simulink model "IP_Core_SS_Switch_and_PWM"  (R2021a)
settings: Solver=VariableStepAuto  StartTime=0.0  StopTime=0.05  RelTol=1e-3
undefined symbols (not defined in the file): f_FPGA_clk, T_FPGA_clk
libraries: hdlsllib x2
(part 1 of 2)
settings Model: Creator=BHK  LastModifiedBy=hoernermi
settings SolverCC: AlgebraicLoopSolver=TrustRegion
settings DataIOCC: ReturnWorkspaceOutputs=off
settings OptimizationCC: BlockReduction=off  ConditionallyExecuteInputs=off  DefaultParameterBehavior=Inlined
settings DebuggingCC: AlgebraicLoopMsg=error  SFMachineParentedDataDiag=warning  ArithmeticOperatorsInVariantConditions=warning
settings HardwareCC: ProdBitPerPointer=32  ProdBitPerSizeT=32  ProdBitPerPtrDiffT=32  ProdLargestAtomicFloat=None  ProdIntDivRoundTo=Undefined  ProdEndianess=Unspecified  ProdWordSize=32  ProdHWDeviceType=ASIC/FPGA->ASIC/FPGA  TargetBitPerPointer=64  TargetBitPerSizeT=64  TargetBitPerPtrDiffT=64  TargetLongLongMode=on  TargetIntDivRoundTo=Zero  TargetEndianess=LittleEndian  TargetWordSize=64  TargetHWDeviceType=Custom Processor->MATLAB Host Computer  ProdEqTarget=off
settings SFSimCC: SimUseLocalCustomCode=off  CustomCodeUndefinedFunction=UseInterfaceOnly
settings RTWCC: RTWUseLocalCustomCode=off

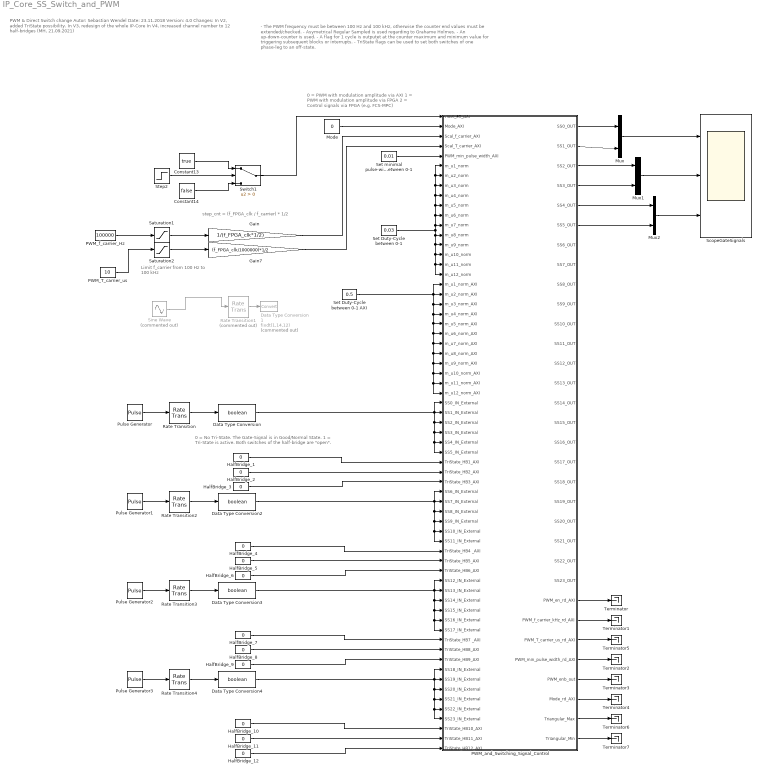
== system IP_Core_SS_Switch_and_PWM ==
  note: 0 = No Tri-State. The Gate-Signal is in Good/Normal State.
      | 1 = Tri-State is active. Both switches of the half-bridge are "open".
  note: PWM & Direct Switch change
      |
      | Autor: Sebastian Wendel
      | Date: 23.11.2018
      | Version: 4.0
      | Changes: In V2, added TriState possibility.
      | In V3, redesign of the whole IP-Core
      | In V4, increased channel number to 12
      | half-bridges (MH, 21.09.2021)
  note: 0 = PWM with modulation amplitude via AXI
      | 1 = PWM with modulation amplitude via FPGA
      | 2 = Control signals via FPGA (e.g. FCS-MPC)
  note: step_cnt = (f_FPGA_clk / f_carrier) * 1/2
  note: Limit f_carrier from
      | 100 Hz to 100 kHz
  note: - The PWM frequency must be between 100 Hz and 100 kHz, otherwise the counter end values must be extended/checked.
      | - Asymetrical Regular Sampled is used regarding to Grahame Holmes.
      | - An up-down-counter is used.
      | - A flag for 1 cycle is outputet at the counter maximum and minimum value for triggering subsequent blocks or interrupts.
      | - TriState flags can be used to set both switches of one phase-leg to an off-state.
  Constant13 : Constant  Value=true  SampleTime=T_FPGA_clk
  Constant14 : Constant  Value=false  SampleTime=T_FPGA_clk
  Data Type Conversion{,2..4} (4 alike) : DataTypeConversion  OutDataTypeStr=boolean
  Data Type Conversion1 : DataTypeConversion  Commented=on  OutDataTypeStr=fixdt(1,14,12)
  Gain : Gain  Gain=1/(f_FPGA_clk*1/2)  OutDataTypeStr=fixdt(0,25,26)
  Gain7 : Gain  Gain=(f_FPGA_clk/1000000)*1/2  OutDataTypeStr=fixdt(0,25,0)
  HalfBridge_{1..12} (12 alike) : Constant  Value=0  OutDataTypeStr=fixdt(0,2,0)  SampleTime=T_FPGA_clk
  Mode : Constant  Value=0  OutDataTypeStr=fixdt(0,2,0)  SampleTime=T_FPGA_clk
  Mux : Mux  Inputs=2
  Mux1 : Mux  Inputs=2
  Mux2 : Mux  Inputs=2
  PWM_T_carrier_us : Constant  Value=10  OutDataTypeStr=uint32  SampleTime=T_FPGA_clk
  PWM_and_Switching_Signal_Control : Subsystem  TreatAsAtomicUnit=on
  PWM_f_carrier_Hz : Constant  Value=100000  OutDataTypeStr=uint32  SampleTime=T_FPGA_clk
  Pulse Generator{,1..3} (4 alike) : DiscretePulseGenerator  PulseType=Time based  Period=0.01  PulseWidth=5
  Rate Transition{,2..4} (4 alike) : RateTransition  OutPortSampleTime=T_FPGA_clk
  Rate Transition1 : RateTransition  Commented=on  OutPortSampleTime=T_FPGA_clk
  Saturation1 : Saturate  UpperLimit=100000  LowerLimit=100
  Saturation2 : Saturate  UpperLimit=10000  LowerLimit=10
  ScopeGateSignals : Scope  NumInputPorts=3
  Set Duty-Cycle between 0-1 : Constant  Value=0.03  OutDataTypeStr=fixdt(1,14,12)  SampleTime=T_FPGA_clk
  Set Duty-Cycle between 0-1 AXI : Constant  Value=0.5  OutDataTypeStr=fixdt(1,14,12)  SampleTime=T_FPGA_clk
  Set minimal pulse-width between 0-1 : Constant  Value=0.01  OutDataTypeStr=fixdt(1,18,16)  SampleTime=T_FPGA_clk
  Sine Wave : Sin  Commented=on  Frequency=500  SampleTime=0
  Step2 : Step  Time=0.002  SampleTime=T_FPGA_clk
  Switch1 : Switch  Criteria=u2 > Threshold
  Terminator{,1..7} (8 alike) : Terminator
  wires:
  Step2/1 -> Switch1/2
  Constant13/1 -> Switch1/1
  Constant14/1 -> Switch1/3
  Switch1/1 -> PWM_and_Switching_Signal_Control/1(PWM_en_AXI)
  Mode/1 -> PWM_and_Switching_Signal_Control/2(Mode_AXI)
  PWM_f_carrier_Hz/1 -> Saturation1/1
  Set minimal pulse-width between 0-1/1 -> PWM_and_Switching_Signal_Control/5(PWM_min_pulse_width_AXI)
  Sine Wave/1 -> Rate Transition1/1
  PWM_and_Switching_Signal_Control/25(PWM_en_rd_AXI) -> Terminator/1
  PWM_and_Switching_Signal_Control/26(PWM_f_carrier_kHz_rd_AXI) -> Terminator1/1
  PWM_and_Switching_Signal_Control/28(PWM_min_pulse_width_rd_AXI) -> Terminator2/1
  PWM_and_Switching_Signal_Control/29(PWM_enb_out) -> Terminator3/1
  PWM_and_Switching_Signal_Control/30(Mode_rd_AXI) -> Terminator4/1
  Set Duty-Cycle between 0-1 AXI/1 -> PWM_and_Switching_Signal_Control/22(m_u5_norm_AXI), PWM_and_Switching_Signal_Control/29(m_u12_norm_AXI), PWM_and_Switching_Signal_Control/28(m_u11_norm_AXI), PWM_and_Switching_Signal_Control/27(m_u10_norm_AXI), PWM_and_Switching_Signal_Control/26(m_u9_norm_AXI), PWM_and_Switching_Signal_Control/25(m_u8_norm_AXI), PWM_and_Switching_Signal_Control/24(m_u7_norm_AXI), PWM_and_Switching_Signal_Control/23(m_u6_norm_AXI), PWM_and_Switching_Signal_Control/21(m_u4_norm_AXI), PWM_and_Switching_Signal_Control/20(m_u3_norm_AXI), PWM_and_Switching_Signal_Control/18(m_u1_norm_AXI), PWM_and_Switching_Signal_Control/19(m_u2_norm_AXI)
  PWM_and_Switching_Signal_Control/1(SS0_OUT) -> Mux/1
  PWM_and_Switching_Signal_Control/2(SS1_OUT) -> Mux/2
  Mux/1 -> ScopeGateSignals/1
  PWM_and_Switching_Signal_Control/3(SS2_OUT) -> Mux1/1
  PWM_and_Switching_Signal_Control/4(SS3_OUT) -> Mux1/2
  PWM_and_Switching_Signal_Control/5(SS4_OUT) -> Mux2/1
  PWM_and_Switching_Signal_Control/6(SS5_OUT) -> Mux2/2
  Mux2/1 -> ScopeGateSignals/3
  Mux1/1 -> ScopeGateSignals/2
  Data Type Conversion/1 -> PWM_and_Switching_Signal_Control/30(SS0_IN_External), PWM_and_Switching_Signal_Control/34(SS4_IN_External), PWM_and_Switching_Signal_Control/35(SS5_IN_External), PWM_and_Switching_Signal_Control/33(SS3_IN_External), PWM_and_Switching_Signal_Control/32(SS2_IN_External), PWM_and_Switching_Signal_Control/31(SS1_IN_External)
  PWM_T_carrier_us/1 -> Saturation2/1
  Rate Transition/1 -> Data Type Conversion/1
  Pulse Generator/1 -> Rate Transition/1
  PWM_and_Switching_Signal_Control/27(PWM_T_carrier_us_rd_AXI) -> Terminator5/1
  PWM_and_Switching_Signal_Control/31(Triangular_Max) -> Terminator6/1
  HalfBridge_3/1 -> PWM_and_Switching_Signal_Control/38(TriState_HB3_AXI)
  HalfBridge_2/1 -> PWM_and_Switching_Signal_Control/37(TriState_HB2_AXI)
  HalfBridge_1/1 -> PWM_and_Switching_Signal_Control/36(TriState_HB1_AXI)
  PWM_and_Switching_Signal_Control/32(Triangular_Min) -> Terminator7/1
  Gain/1 -> PWM_and_Switching_Signal_Control/3(Scal_f_carrier_AXI)
  Gain7/1 -> PWM_and_Switching_Signal_Control/4(Scal_T_carrier_AXI)
  Saturation1/1 -> Gain/1
  Saturation2/1 -> Gain7/1
  Rate Transition1/1 -> Data Type Conversion1/1
  Set Duty-Cycle between 0-1/1 -> PWM_and_Switching_Signal_Control/6(m_u1_norm), PWM_and_Switching_Signal_Control/7(m_u2_norm), PWM_and_Switching_Signal_Control/8(m_u3_norm), PWM_and_Switching_Signal_Control/9(m_u4_norm), PWM_and_Switching_Signal_Control/10(m_u5_norm), PWM_and_Switching_Signal_Control/11(m_u6_norm), PWM_and_Switching_Signal_Control/12(m_u7_norm), PWM_and_Switching_Signal_Control/17(m_u12_norm), PWM_and_Switching_Signal_Control/16(m_u11_norm), PWM_and_Switching_Signal_Control/15(m_u10_norm), PWM_and_Switching_Signal_Control/14(m_u9_norm), PWM_and_Switching_Signal_Control/13(m_u8_norm)
  HalfBridge_5/1 -> PWM_and_Switching_Signal_Control/46(TriState_HB5_AXI)
  HalfBridge_6/1 -> PWM_and_Switching_Signal_Control/47(TriState_HB6_AXI)
  HalfBridge_4/1 -> PWM_and_Switching_Signal_Control/45(TriState_HB4	_AXI)
  HalfBridge_8/1 -> PWM_and_Switching_Signal_Control/55(TriState_HB8_AXI)
  HalfBridge_9/1 -> PWM_and_Switching_Signal_Control/56(TriState_HB9_AXI)
  HalfBridge_7/1 -> PWM_and_Switching_Signal_Control/54(TriState_HB7	_AXI)
  HalfBridge_11/1 -> PWM_and_Switching_Signal_Control/64(TriState_HB11_AXI)
  HalfBridge_12/1 -> PWM_and_Switching_Signal_Control/65(TriState_HB12_AXI)
  HalfBridge_10/1 -> PWM_and_Switching_Signal_Control/63(TriState_HB10_AXI)
  Rate Transition2/1 -> Data Type Conversion2/1
  Pulse Generator1/1 -> Rate Transition2/1
  Data Type Conversion2/1 -> PWM_and_Switching_Signal_Control/40(SS7_IN_External), PWM_and_Switching_Signal_Control/39(SS6_IN_External), PWM_and_Switching_Signal_Control/41(SS8_IN_External), PWM_and_Switching_Signal_Control/42(SS9_IN_External), PWM_and_Switching_Signal_Control/43(SS10_IN_External), PWM_and_Switching_Signal_Control/44(SS11_IN_External)
  Rate Transition3/1 -> Data Type Conversion3/1
  Pulse Generator2/1 -> Rate Transition3/1
  Data Type Conversion3/1 -> PWM_and_Switching_Signal_Control/48(SS12_IN_External), PWM_and_Switching_Signal_Control/49(SS13_IN_External), PWM_and_Switching_Signal_Control/50(SS14_IN_External), PWM_and_Switching_Signal_Control/51(SS15_IN_External), PWM_and_Switching_Signal_Control/53(SS17_IN_External), PWM_and_Switching_Signal_Control/52(SS16_IN_External)
  Rate Transition4/1 -> Data Type Conversion4/1
  Pulse Generator3/1 -> Rate Transition4/1
  Data Type Conversion4/1 -> PWM_and_Switching_Signal_Control/58(SS19_IN_External), PWM_and_Switching_Signal_Control/57(SS18_IN_External), PWM_and_Switching_Signal_Control/59(SS20_IN_External), PWM_and_Switching_Signal_Control/60(SS21_IN_External), PWM_and_Switching_Signal_Control/61(SS22_IN_External), PWM_and_Switching_Signal_Control/62(SS23_IN_External)

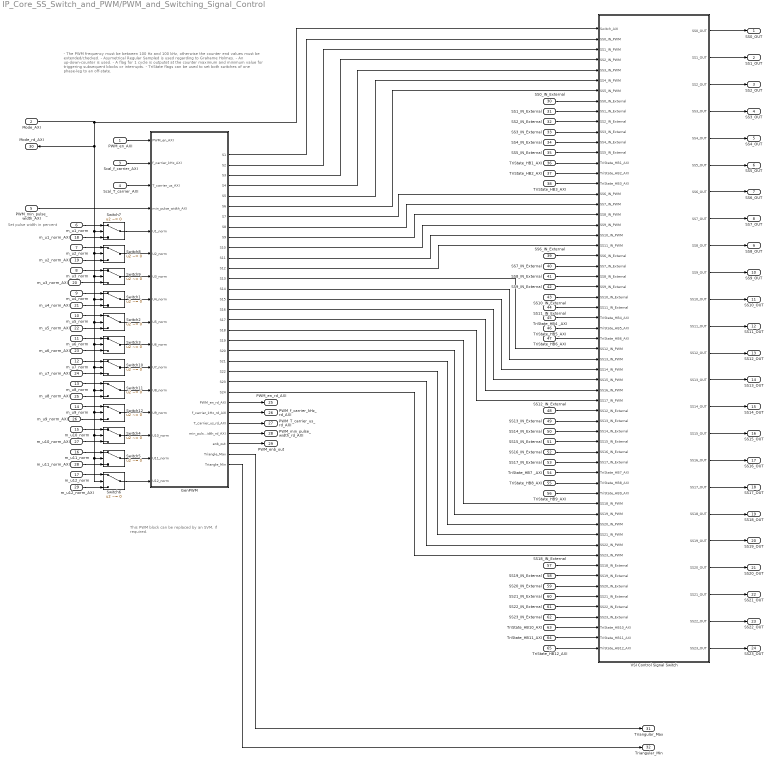
== system IP_Core_SS_Switch_and_PWM/PWM_and_Switching_Signal_Control ==
  note: This PWM block can be replaced by an SVM,
      | if required.
  note: - The PWM frequency must be between 100 Hz and 100 kHz, otherwise the counter end values must be extended/checked.
      | - Asymetrical Regular Sampled is used regarding to Grahame Holmes.
      | - An up-down-counter is used.
      | - A flag for 1 cycle is outputet at the counter maximum and minimum value for triggering subsequent blocks or interrupts.
      | - TriState flags can be used to set both switches of one phase-leg to an off-state.
  note: Set pulse width in percent
  PWM_en_AXI : Inport
  Mode_AXI : Inport  Port=2
  Scal_f_carrier_AXI : Inport  Port=3
  Scal_T_carrier_AXI : Inport  Port=4
  PWM_min_pulse_width_AXI : Inport  Port=5
  m_u1_norm : Inport  Port=6
  m_u2_norm : Inport  Port=7
  m_u3_norm : Inport  Port=8
  m_u4_norm : Inport  Port=9
  m_u5_norm : Inport  Port=10
  m_u6_norm : Inport  Port=11
  m_u7_norm : Inport  Port=12
  m_u8_norm : Inport  Port=13
  m_u9_norm : Inport  Port=14
  m_u10_norm : Inport  Port=15
  m_u11_norm : Inport  Port=16
  m_u12_norm : Inport  Port=17
  m_u1_norm_AXI : Inport  Port=18
  m_u2_norm_AXI : Inport  Port=19
  m_u3_norm_AXI : Inport  Port=20
  m_u4_norm_AXI : Inport  Port=21
  m_u5_norm_AXI : Inport  Port=22
  m_u6_norm_AXI : Inport  Port=23
  m_u7_norm_AXI : Inport  Port=24
  m_u8_norm_AXI : Inport  Port=25
  m_u9_norm_AXI : Inport  Port=26
  m_u10_norm_AXI : Inport  Port=27
  m_u11_norm_AXI : Inport  Port=28
  m_u12_norm_AXI : Inport  Port=29
  SS0_IN_External : Inport  Port=30
  SS1_IN_External : Inport  Port=31
  SS2_IN_External : Inport  Port=32
  SS3_IN_External : Inport  Port=33
  SS4_IN_External : Inport  Port=34
  SS5_IN_External : Inport  Port=35
  TriState_HB1_AXI : Inport  Port=36
  TriState_HB2_AXI : Inport  Port=37
  TriState_HB3_AXI : Inport  Port=38
  SS6_IN_External : Inport  Port=39
  SS7_IN_External : Inport  Port=40
  SS8_IN_External : Inport  Port=41
  SS9_IN_External : Inport  Port=42
  SS10_IN_External : Inport  Port=43
  SS11_IN_External : Inport  Port=44
  TriState_HB4	_AXI : Inport  Port=45
  TriState_HB5_AXI : Inport  Port=46
  TriState_HB6_AXI : Inport  Port=47
  SS12_IN_External : Inport  Port=48
  SS13_IN_External : Inport  Port=49
  SS14_IN_External : Inport  Port=50
  SS15_IN_External : Inport  Port=51
  SS16_IN_External : Inport  Port=52
  SS17_IN_External : Inport  Port=53
  TriState_HB7	_AXI : Inport  Port=54
  TriState_HB8_AXI : Inport  Port=55
  TriState_HB9_AXI : Inport  Port=56
  SS18_IN_External : Inport  Port=57
  SS19_IN_External : Inport  Port=58
  SS20_IN_External : Inport  Port=59
  SS21_IN_External : Inport  Port=60
  SS22_IN_External : Inport  Port=61
  SS23_IN_External : Inport  Port=62
  TriState_HB10_AXI : Inport  Port=63
  TriState_HB11_AXI : Inport  Port=64
  TriState_HB12_AXI : Inport  Port=65
  GenPWM : Subsystem  TreatAsAtomicUnit=on
  Switch{1..12} (12 alike) : Switch  Criteria=u2 ~= 0
  VSI Control Signal Switch : Subsystem
  SS0_OUT : Outport  VectorParamsAs1DForOutWhenUnconnected=off
  SS1_OUT : Outport  Port=2  VectorParamsAs1DForOutWhenUnconnected=off
  SS2_OUT : Outport  Port=3  VectorParamsAs1DForOutWhenUnconnected=off
  SS3_OUT : Outport  Port=4  VectorParamsAs1DForOutWhenUnconnected=off
  SS4_OUT : Outport  Port=5  VectorParamsAs1DForOutWhenUnconnected=off
  SS5_OUT : Outport  Port=6  VectorParamsAs1DForOutWhenUnconnected=off
  SS6_OUT : Outport  Port=7  VectorParamsAs1DForOutWhenUnconnected=off
  SS7_OUT : Outport  Port=8  VectorParamsAs1DForOutWhenUnconnected=off
  SS8_OUT : Outport  Port=9  VectorParamsAs1DForOutWhenUnconnected=off
  SS9_OUT : Outport  Port=10  VectorParamsAs1DForOutWhenUnconnected=off
  SS10_OUT : Outport  Port=11  VectorParamsAs1DForOutWhenUnconnected=off
  SS11_OUT : Outport  Port=12  VectorParamsAs1DForOutWhenUnconnected=off
  SS12_OUT : Outport  Port=13  VectorParamsAs1DForOutWhenUnconnected=off
  SS13_OUT : Outport  Port=14  VectorParamsAs1DForOutWhenUnconnected=off
  SS14_OUT : Outport  Port=15  VectorParamsAs1DForOutWhenUnconnected=off
  SS15_OUT : Outport  Port=16  VectorParamsAs1DForOutWhenUnconnected=off
  SS16_OUT : Outport  Port=17  VectorParamsAs1DForOutWhenUnconnected=off
  SS17_OUT : Outport  Port=18  VectorParamsAs1DForOutWhenUnconnected=off
  SS18_OUT : Outport  Port=19  VectorParamsAs1DForOutWhenUnconnected=off
  SS19_OUT : Outport  Port=20  VectorParamsAs1DForOutWhenUnconnected=off
  SS20_OUT : Outport  Port=21  VectorParamsAs1DForOutWhenUnconnected=off
  SS21_OUT : Outport  Port=22  VectorParamsAs1DForOutWhenUnconnected=off
  SS22_OUT : Outport  Port=23  VectorParamsAs1DForOutWhenUnconnected=off
  SS23_OUT : Outport  Port=24  VectorParamsAs1DForOutWhenUnconnected=off
  PWM_en_rd_AXI : Outport  Port=25  VectorParamsAs1DForOutWhenUnconnected=off
  PWM_f_carrier_kHz_rd_AXI : Outport  Port=26  VectorParamsAs1DForOutWhenUnconnected=off
  PWM_T_carrier_us_rd_AXI : Outport  Port=27  VectorParamsAs1DForOutWhenUnconnected=off
  PWM_min_pulse_width_rd_AXI : Outport  Port=28  VectorParamsAs1DForOutWhenUnconnected=off
  PWM_enb_out : Outport  Port=29  VectorParamsAs1DForOutWhenUnconnected=off
  Mode_rd_AXI : Outport  Port=30  VectorParamsAs1DForOutWhenUnconnected=off
  Triangular_Max : Outport  Port=31  VectorParamsAs1DForOutWhenUnconnected=off
  Triangular_Min : Outport  Port=32  VectorParamsAs1DForOutWhenUnconnected=off
  wires:
  VSI Control Signal Switch/1(SS0_OUT) -> SS0_OUT/1
  GenPWM/4(S4) -> VSI Control Signal Switch/5(SS3_IN_PWM)
  Scal_f_carrier_AXI/1 -> GenPWM/2(f_carrier_kHz_AXI)
  GenPWM/2(S2) -> VSI Control Signal Switch/3(SS1_IN_PWM)
  SS1_IN_External/1 -> VSI Control Signal Switch/9(SS1_IN_External)
  GenPWM/3(S3) -> VSI Control Signal Switch/4(SS2_IN_PWM)
  GenPWM/5(S5) -> VSI Control Signal Switch/6(SS4_IN_PWM)
  GenPWM/6(S6) -> VSI Control Signal Switch/7(SS5_IN_PWM)
  VSI Control Signal Switch/6(SS5_OUT) -> SS5_OUT/1
  GenPWM/1(S1) -> VSI Control Signal Switch/2(SS0_IN_PWM)
  GenPWM/29(enb_out) -> PWM_enb_out/1
  VSI Control Signal Switch/3(SS2_OUT) -> SS2_OUT/1
  SS3_IN_External/1 -> VSI Control Signal Switch/11(SS3_IN_External)
  SS0_IN_External/1 -> VSI Control Signal Switch/8(SS0_IN_External)
  VSI Control Signal Switch/2(SS1_OUT) -> SS1_OUT/1
  SS4_IN_External/1 -> VSI Control Signal Switch/12(SS4_IN_External)
  PWM_en_AXI/1 -> GenPWM/1(PWM_en_AXI)
  SS5_IN_External/1 -> VSI Control Signal Switch/13(SS5_IN_External)
  VSI Control Signal Switch/5(SS4_OUT) -> SS4_OUT/1
  PWM_min_pulse_width_AXI/1 -> GenPWM/4(min_pulse_width_AXI)
  SS2_IN_External/1 -> VSI Control Signal Switch/10(SS2_IN_External)
  VSI Control Signal Switch/4(SS3_OUT) -> SS3_OUT/1
  Switch9/1 -> GenPWM/7(U3_norm)
  m_u1_norm_AXI/1 -> Switch7/3
  m_u1_norm/1 -> Switch7/1
  m_u2_norm/1 -> Switch8/1
  m_u2_norm_AXI/1 -> Switch8/3
  m_u3_norm/1 -> Switch9/1
  m_u3_norm_AXI/1 -> Switch9/3
  GenPWM/25(PWM_en_rd_AXI) -> PWM_en_rd_AXI/1
  GenPWM/26(f_carrier_kHz_rd_AXI) -> PWM_f_carrier_kHz_rd_AXI/1
  GenPWM/28(min_pulse_width_rd_AXI) -> PWM_min_pulse_width_rd_AXI/1
  GenPWM/27(T_carrier_us_rd_AXI) -> PWM_T_carrier_us_rd_AXI/1
  Switch8/1 -> GenPWM/6(U2_norm)
  Switch7/1 -> GenPWM/5(U1_norm)
  Scal_T_carrier_AXI/1 -> GenPWM/3(T_carrier_us_AXI)
  GenPWM/30(Triangle_Max) -> Triangular_Max/1
  TriState_HB1_AXI/1 -> VSI Control Signal Switch/14(TriState_HB1_AXI)
  TriState_HB2_AXI/1 -> VSI Control Signal Switch/15(TriState_HB2_AXI)
  TriState_HB3_AXI/1 -> VSI Control Signal Switch/16(TriState_HB3_AXI)
  GenPWM/31(Triangle_Min) -> Triangular_Min/1
  GenPWM/7(S7) -> VSI Control Signal Switch/17(SS6_IN_PWM)
  GenPWM/8(S8) -> VSI Control Signal Switch/18(SS7_IN_PWM)
  GenPWM/9(S9) -> VSI Control Signal Switch/19(SS8_IN_PWM)
  GenPWM/10(S10) -> VSI Control Signal Switch/20(SS9_IN_PWM)
  GenPWM/11(S11) -> VSI Control Signal Switch/21(SS10_IN_PWM)
  GenPWM/12(S12) -> VSI Control Signal Switch/22(SS11_IN_PWM)
  SS6_IN_External/1 -> VSI Control Signal Switch/23(SS6_IN_External)
  TriState_HB6_AXI/1 -> VSI Control Signal Switch/31(TriState_HB6_AXI)
  SS10_IN_External/1 -> VSI Control Signal Switch/27(SS10_IN_External)
  TriState_HB5_AXI/1 -> VSI Control Signal Switch/30(TriState_HB5_AXI)
  SS11_IN_External/1 -> VSI Control Signal Switch/28(SS11_IN_External)
  SS8_IN_External/1 -> VSI Control Signal Switch/25(SS8_IN_External)
  SS9_IN_External/1 -> VSI Control Signal Switch/26(SS9_IN_External)
  SS7_IN_External/1 -> VSI Control Signal Switch/24(SS7_IN_External)
  TriState_HB4	_AXI/1 -> VSI Control Signal Switch/29(TriState_HB4_AXI)
  GenPWM/13(S13) -> VSI Control Signal Switch/32(SS12_IN_PWM)
  GenPWM/14(S14) -> VSI Control Signal Switch/33(SS13_IN_PWM)
  GenPWM/15(S15) -> VSI Control Signal Switch/34(SS14_IN_PWM)
  GenPWM/16(S16) -> VSI Control Signal Switch/35(SS15_IN_PWM)
  GenPWM/17(S17) -> VSI Control Signal Switch/36(SS16_IN_PWM)
  GenPWM/18(S18) -> VSI Control Signal Switch/37(SS17_IN_PWM)
  SS16_IN_External/1 -> VSI Control Signal Switch/42(SS16_IN_External)
  SS14_IN_External/1 -> VSI Control Signal Switch/40(SS14_IN_External)
  SS13_IN_External/1 -> VSI Control Signal Switch/39(SS13_IN_External)
  TriState_HB9_AXI/1 -> VSI Control Signal Switch/46(TriState_HB9_AXI)
  SS15_IN_External/1 -> VSI Control Signal Switch/41(SS15_IN_External)
  TriState_HB8_AXI/1 -> VSI Control Signal Switch/45(TriState_HB8_AXI)
  SS12_IN_External/1 -> VSI Control Signal Switch/38(SS12_IN_External)
  SS17_IN_External/1 -> VSI Control Signal Switch/43(SS17_IN_External)
  TriState_HB7	_AXI/1 -> VSI Control Signal Switch/44(TriState_HB7_AXI)
  GenPWM/19(S19) -> VSI Control Signal Switch/47(SS18_IN_PWM)
  GenPWM/20(S20) -> VSI Control Signal Switch/48(SS19_IN_PWM)
  GenPWM/21(S21) -> VSI Control Signal Switch/49(SS20_IN_PWM)
  GenPWM/22(S22) -> VSI Control Signal Switch/50(SS21_IN_PWM)
  GenPWM/23(S23) -> VSI Control Signal Switch/51(SS22_IN_PWM)
  GenPWM/24(S24) -> VSI Control Signal Switch/52(SS23_IN_PWM)
  TriState_HB10_AXI/1 -> VSI Control Signal Switch/59(TriState_HB10_AXI)
  TriState_HB12_AXI/1 -> VSI Control Signal Switch/61(TriState_HB12_AXI)
  SS21_IN_External/1 -> VSI Control Signal Switch/56(SS21_IN_External)
  SS22_IN_External/1 -> VSI Control Signal Switch/57(SS22_IN_External)
  SS23_IN_External/1 -> VSI Control Signal Switch/58(SS23_IN_External)
  SS18_IN_External/1 -> VSI Control Signal Switch/53(SS18_IN_External)
  TriState_HB11_AXI/1 -> VSI Control Signal Switch/60(TriState_HB11_AXI)
  SS20_IN_External/1 -> VSI Control Signal Switch/55(SS20_IN_External)
  SS19_IN_External/1 -> VSI Control Signal Switch/54(SS19_IN_External)
  VSI Control Signal Switch/11(SS10_OUT) -> SS10_OUT/1
  VSI Control Signal Switch/8(SS7_OUT) -> SS7_OUT/1
  VSI Control Signal Switch/7(SS6_OUT) -> SS6_OUT/1
  VSI Control Signal Switch/10(SS9_OUT) -> SS9_OUT/1
  VSI Control Signal Switch/12(SS11_OUT) -> SS11_OUT/1
  VSI Control Signal Switch/9(SS8_OUT) -> SS8_OUT/1
  VSI Control Signal Switch/21(SS20_OUT) -> SS20_OUT/1
  VSI Control Signal Switch/19(SS18_OUT) -> SS18_OUT/1
  VSI Control Signal Switch/22(SS21_OUT) -> SS21_OUT/1
  VSI Control Signal Switch/20(SS19_OUT) -> SS19_OUT/1
  VSI Control Signal Switch/17(SS16_OUT) -> SS16_OUT/1
  VSI Control Signal Switch/14(SS13_OUT) -> SS13_OUT/1
  VSI Control Signal Switch/16(SS15_OUT) -> SS15_OUT/1
  VSI Control Signal Switch/13(SS12_OUT) -> SS12_OUT/1
  VSI Control Signal Switch/23(SS22_OUT) -> SS22_OUT/1
  VSI Control Signal Switch/18(SS17_OUT) -> SS17_OUT/1
  VSI Control Signal Switch/24(SS23_OUT) -> SS23_OUT/1
  VSI Control Signal Switch/15(SS14_OUT) -> SS14_OUT/1
  Switch2/1 -> GenPWM/9(U5_norm)
  m_u5_norm_AXI/1 -> Switch2/3
  Switch3/1 -> GenPWM/10(U6_norm)
  m_u4_norm_AXI/1 -> Switch1/3
  m_u4_norm/1 -> Switch1/1
  m_u6_norm/1 -> Switch3/1
  m_u6_norm_AXI/1 -> Switch3/3
  m_u5_norm/1 -> Switch2/1
  Switch1/1 -> GenPWM/8(U4_norm)
  m_u11_norm/1 -> Switch5/1
  m_u12_norm_AXI/1 -> Switch6/3
  m_u12_norm/1 -> Switch6/1
  m_u10_norm/1 -> Switch4/1
  m_u11_norm_AXI/1 -> Switch5/3
  m_u10_norm_AXI/1 -> Switch4/3
  Switch6/1 -> GenPWM/16(U12_norm)
  Switch5/1 -> GenPWM/15(U11_norm)
  Switch4/1 -> GenPWM/14(U10_norm)
  Switch11/1 -> GenPWM/12(U8_norm)
  m_u8_norm_AXI/1 -> Switch11/3
  Switch12/1 -> GenPWM/13(U9_norm)
  m_u7_norm_AXI/1 -> Switch10/3
  m_u7_norm/1 -> Switch10/1
  m_u9_norm/1 -> Switch12/1
  Mode_AXI/1 -> Mode_rd_AXI/1, Switch1/2, Switch4/2, Switch6/2, Switch5/2, Switch12/2, Switch11/2, Switch10/2, Switch3/2, Switch2/2, Switch9/2, Switch8/2, Switch7/2, VSI Control Signal Switch/1(Switch_AXI)
  m_u9_norm_AXI/1 -> Switch12/3
  m_u8_norm/1 -> Switch11/1
  Switch10/1 -> GenPWM/11(U7_norm)

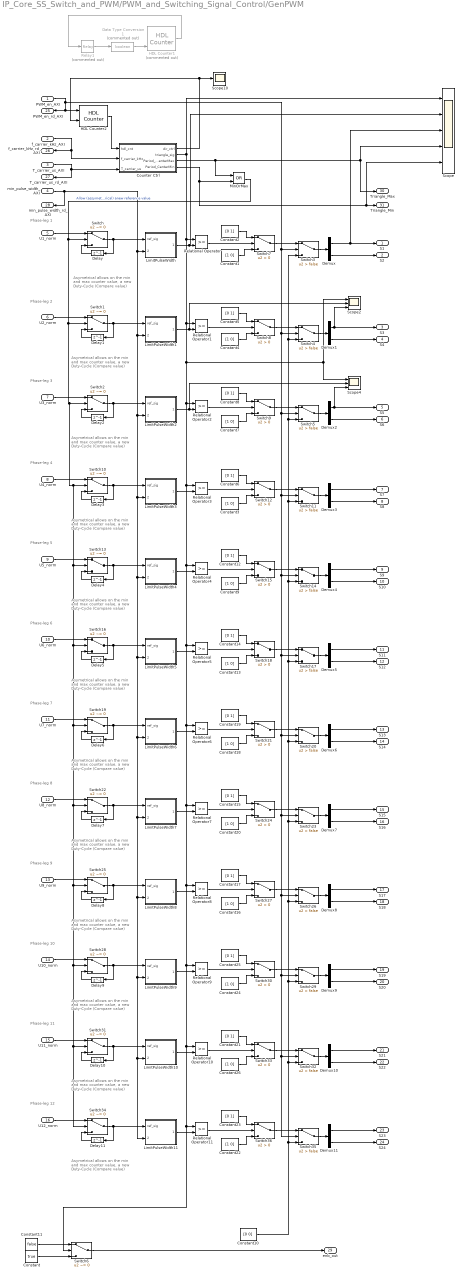
== system IP_Core_SS_Switch_and_PWM/PWM_and_Switching_Signal_Control/GenPWM ==
  note: Asymetrical allows on the min
      |  and max counter value, a new
      |  Duty-Cycle (Compare value)
  note: Phase-leg 1
  note: Phase-leg 2
  note: Phase-leg 3
  note: Asymetrical allows on the min
      |  and max counter value, a new
      |  Duty-Cycle (Compare value)
  note: Asymetrical allows on the min
      |  and max counter value, a new
      |  Duty-Cycle (Compare value)
  note: Phase-leg 4
  note: Asymetrical allows on the min
      |  and max counter value, a new
      |  Duty-Cycle (Compare value)
  note: Phase-leg 5
  note: Asymetrical allows on the min
      |  and max counter value, a new
      |  Duty-Cycle (Compare value)
  note: Phase-leg 6
  note: Asymetrical allows on the min
      |  and max counter value, a new
      |  Duty-Cycle (Compare value)
  note: Asymetrical allows on the min
      |  and max counter value, a new
      |  Duty-Cycle (Compare value)
  note: Phase-leg 9
  note: Asymetrical allows on the min
      |  and max counter value, a new
      |  Duty-Cycle (Compare value)
  note: Phase-leg 8
  note: Asymetrical allows on the min
      |  and max counter value, a new
      |  Duty-Cycle (Compare value)
  note: Phase-leg 7
  note: Asymetrical allows on the min
      |  and max counter value, a new
      |  Duty-Cycle (Compare value)
  note: Phase-leg 12
  note: Asymetrical allows on the min
      |  and max counter value, a new
      |  Duty-Cycle (Compare value)
  note: Phase-leg 11
  note: Asymetrical allows on the min
      |  and max counter value, a new
      |  Duty-Cycle (Compare value)
  note: Phase-leg 10
  PWM_en_AXI : Inport
  f_carrier_kHz_AXI : Inport  Port=2
  T_carrier_us_AXI : Inport  Port=3
  min_pulse_width_AXI : Inport  Port=4
  U1_norm : Inport  Port=5
  U2_norm : Inport  Port=6
  U3_norm : Inport  Port=7
  U4_norm : Inport  Port=8
  U5_norm : Inport  Port=9
  U6_norm : Inport  Port=10
  U7_norm : Inport  Port=11
  U8_norm : Inport  Port=12
  U9_norm : Inport  Port=13
  U10_norm : Inport  Port=14
  U11_norm : Inport  Port=15
  U12_norm : Inport  Port=16
  Constant : Constant  Value=true  SampleTime=T_FPGA_clk
  Constant{1,3..4,7,9,13,16,18,20,22,24,26} (12 alike) : Constant  Value=[1 0]  OutDataTypeStr=fixdt(0,1,0)  SampleTime=T_FPGA_clk
  Constant10 : Constant  Value=[0 0]  OutDataTypeStr=fixdt(0,1,0)  SampleTime=T_FPGA_clk
  Constant11 : Constant  Value=false  SampleTime=T_FPGA_clk
  Constant{2,5..6,8,12,14..15,17,19,21,23,25} (12 alike) : Constant  Value=[0 1]  OutDataTypeStr=fixdt(0,1,0)  SampleTime=T_FPGA_clk
  Counter Ctrl : Subsystem
  Data Type Conversion1 : DataTypeConversion  Commented=on  OutDataTypeStr=boolean
  Delay{,1..11} (12 alike) : Delay  DelayLength=1
  Demux{,1..11} (12 alike) : Demux  Outputs=2
  HDL Counter1 : hdlsllib/Sources/HDL Counter  Commented=on  CountType=Free running  CountInit=0  CountStep=1  CountMax=100  CountFromType=Initial value  CountFrom=0  CountResetPort=on  CountLoadPort=off  CountEnbPort=on  CountDirPort=on  CountHitOutputPort=off  CountDataType=Signed  CountWordLen=8  CountFracLen=0  CountSampTime=Ts
  HDL Counter2 : hdlsllib/Sources/HDL Counter  CountType=Free running  CountInit=0  CountStep=1  CountMax=100  CountFromType=Initial value  CountFrom=0  CountResetPort=off  CountLoadPort=off  CountEnbPort=on  CountDirPort=on  CountHitOutputPort=off  CountDataType=Unsigned  CountWordLen=20  CountFracLen=0  CountSampTime=1
  LimitPulseWidth : Subsystem
  LimitPulseWidth1 : Subsystem
  LimitPulseWidth10 : Subsystem
  LimitPulseWidth11 : Subsystem
  LimitPulseWidth2 : Subsystem
  LimitPulseWidth3 : Subsystem
  LimitPulseWidth4 : Subsystem
  LimitPulseWidth5 : Subsystem
  LimitPulseWidth6 : Subsystem
  LimitPulseWidth7 : Subsystem
  LimitPulseWidth8 : Subsystem
  LimitPulseWidth9 : Subsystem
  MinOrMax : Logic  Operator=OR  AllPortsSameDT=off  OutDataTypeStr=boolean
  Relational Operator{,1..11} (12 alike) : RelationalOperator  OutDataTypeStr=boolean  RndMeth=Nearest
  Relay1 : Relay  Commented=on  OnSwitchValue=100  OffSwitchValue=0  OnOutputValue=0  OffOutputValue=1
  Scope : Scope  NumInputPorts=5
  Scope10 : Scope
  Scope2 : Scope  NumInputPorts=3
  Scope4 : Scope  NumInputPorts=3
  Switch : Switch  Criteria=u2 ~= 0  Threshold=1
  Switch{1..2,6,10,13,16,19,22,25,28,31,34} (12 alike) : Switch  Criteria=u2 ~= 0
  Switch{3..5,11,14,17,20,23,26,29,32,35} (12 alike) : Switch  Criteria=u2 > Threshold  Threshold=false
  Switch{7..9,12,15,18,21,24,27,30,33,36} (12 alike) : Switch  Criteria=u2 > Threshold
  S1 : Outport  VectorParamsAs1DForOutWhenUnconnected=off
  S2 : Outport  Port=2  VectorParamsAs1DForOutWhenUnconnected=off
  S3 : Outport  Port=3  VectorParamsAs1DForOutWhenUnconnected=off
  S4 : Outport  Port=4  VectorParamsAs1DForOutWhenUnconnected=off
  S5 : Outport  Port=5  VectorParamsAs1DForOutWhenUnconnected=off
  S6 : Outport  Port=6  VectorParamsAs1DForOutWhenUnconnected=off
  S7 : Outport  Port=7  VectorParamsAs1DForOutWhenUnconnected=off
  S8 : Outport  Port=8  VectorParamsAs1DForOutWhenUnconnected=off
  S9 : Outport  Port=9  VectorParamsAs1DForOutWhenUnconnected=off
  S10 : Outport  Port=10  VectorParamsAs1DForOutWhenUnconnected=off
  S11 : Outport  Port=11  VectorParamsAs1DForOutWhenUnconnected=off
  S12 : Outport  Port=12  VectorParamsAs1DForOutWhenUnconnected=off
  S13 : Outport  Port=13  VectorParamsAs1DForOutWhenUnconnected=off
  S14 : Outport  Port=14  VectorParamsAs1DForOutWhenUnconnected=off
  S15 : Outport  Port=15  VectorParamsAs1DForOutWhenUnconnected=off
  S16 : Outport  Port=16  VectorParamsAs1DForOutWhenUnconnected=off
  S17 : Outport  Port=17  VectorParamsAs1DForOutWhenUnconnected=off
  S18 : Outport  Port=18  VectorParamsAs1DForOutWhenUnconnected=off
  S19 : Outport  Port=19  VectorParamsAs1DForOutWhenUnconnected=off
  S20 : Outport  Port=20  VectorParamsAs1DForOutWhenUnconnected=off
  S21 : Outport  Port=21  VectorParamsAs1DForOutWhenUnconnected=off
  S22 : Outport  Port=22  VectorParamsAs1DForOutWhenUnconnected=off
  S23 : Outport  Port=23  VectorParamsAs1DForOutWhenUnconnected=off
  S24 : Outport  Port=24  VectorParamsAs1DForOutWhenUnconnected=off
  PWM_en_rd_AXI : Outport  Port=25  VectorParamsAs1DForOutWhenUnconnected=off
  f_carrier_kHz_rd_AXI : Outport  Port=26  VectorParamsAs1DForOutWhenUnconnected=off
  T_carrier_us_rd_AXI : Outport  Port=27  VectorParamsAs1DForOutWhenUnconnected=off
  min_pulse_width_rd_AXI : Outport  Port=28  VectorParamsAs1DForOutWhenUnconnected=off
  enb_out : Outport  Port=29  VectorParamsAs1DForOutWhenUnconnected=off
  Triangle_Max : Outport  Port=30  VectorParamsAs1DForOutWhenUnconnected=off
  Triangle_Min : Outport  Port=31  VectorParamsAs1DForOutWhenUnconnected=off
  wires:
  Constant7/1 -> Switch9/3
  Demux2/2 -> S6/1
  Constant8/1 -> Switch9/1
  Relational Operator2/1 -> Switch9/2
  Switch9/1 -> Switch5/1
  Demux/2 -> S2/1
  Relational Operator/1 -> Switch7/2
  Demux1/2 -> S4/1
  Constant5/1 -> Switch8/1
  Relational Operator1/1 -> Switch8/2
  Constant4/1 -> Switch8/3
  Constant1/1 -> Switch7/3
  Constant2/1 -> Switch7/1
  LimitPulseWidth/1(ref_sig_limit) -> Scope/2, Relational Operator/2
  LimitPulseWidth1/1(ref_sig_limit) -> Scope2/2, Relational Operator1/2
  LimitPulseWidth2/1(ref_sig_limit) -> Scope4/2, Relational Operator2/2
  Delay/1 -> Switch/3
  Delay1/1 -> Switch1/3
  Delay2/1 -> Switch2/3
  Switch5/1 -> Demux2/1
  Switch8/1 -> Switch4/1
  Switch4/1 -> Demux1/1
  Switch3/1 -> Demux/1
  U1_norm/1 -> Switch/1
  U3_norm/1 -> Switch2/1
  U2_norm/1 -> Switch1/1
  Counter Ctrl/1(dir_ctrl) -> HDL Counter2/2, Scope10/1
  HDL Counter2/1 -> Counter Ctrl/1(hdl_cnt)
  f_carrier_kHz_AXI/1 -> f_carrier_kHz_rd_AXI/1, Counter Ctrl/2(f_carrier_kHz)
  Relay1/1 -> Data Type Conversion1/1
  Data Type Conversion1/1 -> HDL Counter1/3
  HDL Counter1/1 -> Relay1/1
  Switch/1 -> Delay/1, LimitPulseWidth/1(ref_sig)
  Switch1/1 -> LimitPulseWidth1/1(ref_sig), Delay1/1
  Switch2/1 -> LimitPulseWidth2/1(ref_sig), Delay2/1
  Demux/1 -> Scope/3, S1/1
  Switch6/1 -> enb_out/1
  Constant11/1 -> Switch6/1
  Constant/1 -> Switch6/3
  Demux1/1 -> Scope2/3, S3/1
  Demux2/1 -> Scope4/3, S5/1
  T_carrier_us_AXI/1 -> T_carrier_us_rd_AXI/1, Counter Ctrl/3(T_carrier_us)
  Switch7/1 -> Switch3/1
  Counter Ctrl/3(Period_CenterMax) -> MinOrMax/1, Triangle_Max/1, Scope/4
  Counter Ctrl/4(Period_CenterMin) -> MinOrMax/2, Scope/5, Triangle_Min/1
  Demux3/1 -> S7/1
  Relational Operator3/1 -> Switch12/2
  Switch10/1 -> LimitPulseWidth3/1(ref_sig), Delay3/1
  Switch11/1 -> Demux3/1
  Delay3/1 -> Switch10/3
  U4_norm/1 -> Switch10/1
  Constant10/1 -> Switch3/3, Switch4/3, Switch5/3, Switch11/3, Switch14/3, Switch17/3, Switch20/3, Switch23/3, Switch26/3, Switch29/3, Switch32/3, Switch35/3
  Constant6/1 -> Switch12/1
  Constant3/1 -> Switch12/3
  Switch12/1 -> Switch11/1
  Demux3/2 -> S8/1
  LimitPulseWidth3/1(ref_sig_limit) -> Relational Operator3/2
  U5_norm/1 -> Switch13/1
  Delay4/1 -> Switch13/3
  LimitPulseWidth4/1(ref_sig_limit) -> Relational Operator4/2
  Switch15/1 -> Switch14/1
  Constant9/1 -> Switch15/3
  Constant12/1 -> Switch15/1
  Counter Ctrl/2(triangle_sig) -> Switch6/2, Relational Operator11/1, Relational Operator10/1, Relational Operator9/1, Relational Operator8/1, Relational Operator7/1, Relational Operator6/1, Relational Operator5/1, Relational Operator4/1, Relational Operator3/1, Relational Operator2/1, Scope2/1, Scope4/1, Relational Operator1/1, Relational Operator/1, Scope/1
  Switch14/1 -> Demux4/1
  Demux4/1 -> S9/1
  Relational Operator4/1 -> Switch15/2
  Switch13/1 -> LimitPulseWidth4/1(ref_sig), Delay4/1
  Demux4/2 -> S10/1
  U6_norm/1 -> Switch16/1
  Delay5/1 -> Switch16/3
  LimitPulseWidth5/1(ref_sig_limit) -> Relational Operator5/2
  Switch18/1 -> Switch17/1
  Constant13/1 -> Switch18/3
  Constant14/1 -> Switch18/1
  Switch17/1 -> Demux5/1
  Demux5/1 -> S11/1
  Relational Operator5/1 -> Switch18/2
  Switch16/1 -> LimitPulseWidth5/1(ref_sig), Delay5/1
  Demux5/2 -> S12/1
  Demux8/2 -> S18/1
  Switch25/1 -> LimitPulseWidth8/1(ref_sig), Delay8/1
  Relational Operator8/1 -> Switch27/2
  Switch26/1 -> Demux8/1
  Demux8/1 -> S17/1
  U7_norm/1 -> Switch19/1
  Constant15/1 -> Switch24/1
  Constant18/1 -> Switch21/3
  Constant19/1 -> Switch21/1
  Switch22/1 -> LimitPulseWidth7/1(ref_sig), Delay7/1
  LimitPulseWidth8/1(ref_sig_limit) -> Relational Operator8/2
  Delay6/1 -> Switch19/3
  Delay7/1 -> Switch22/3
  U8_norm/1 -> Switch22/1
  Constant20/1 -> Switch24/3
  Switch21/1 -> Switch20/1
  LimitPulseWidth7/1(ref_sig_limit) -> Relational Operator7/2
  Switch24/1 -> Switch23/1
  Switch19/1 -> LimitPulseWidth6/1(ref_sig), Delay6/1
  Relational Operator7/1 -> Switch24/2
  Demux6/1 -> S13/1
  Relational Operator6/1 -> Switch21/2
  U9_norm/1 -> Switch25/1
  Delay8/1 -> Switch25/3
  Demux7/2 -> S16/1
  Constant17/1 -> Switch27/1
  Switch20/1 -> Demux6/1
  LimitPulseWidth6/1(ref_sig_limit) -> Relational Operator6/2
  Switch23/1 -> Demux7/1
  Constant16/1 -> Switch27/3
  Switch27/1 -> Switch26/1
  Demux6/2 -> S14/1
  Demux7/1 -> S15/1
  Demux11/2 -> S24/1
  MinOrMax/1 -> Switch1/2, Switch34/2, Switch31/2, Switch28/2, Switch25/2, Switch22/2, Switch19/2, Switch16/2, Switch13/2, Switch10/2, Switch2/2, Switch/2  "Allow (assymetrical) anew reference value"
  min_pulse_width_AXI/1 -> LimitPulseWidth/2(min_pulse_width), LimitPulseWidth4/2(min_pulse_width), LimitPulseWidth11/2(min_pulse_width), LimitPulseWidth10/2(min_pulse_width), LimitPulseWidth9/2(min_pulse_width), LimitPulseWidth8/2(min_pulse_width), LimitPulseWidth7/2(min_pulse_width), LimitPulseWidth6/2(min_pulse_width), LimitPulseWidth5/2(min_pulse_width), LimitPulseWidth3/2(min_pulse_width), LimitPulseWidth2/2(min_pulse_width), LimitPulseWidth1/2(min_pulse_width), min_pulse_width_rd_AXI/1
  Switch34/1 -> LimitPulseWidth11/1(ref_sig), Delay11/1
  Relational Operator11/1 -> Switch36/2
  Switch35/1 -> Demux11/1
  Demux11/1 -> S23/1
  U10_norm/1 -> Switch28/1
  Constant21/1 -> Switch33/1
  Constant24/1 -> Switch30/3
  Constant25/1 -> Switch30/1
  Switch31/1 -> LimitPulseWidth10/1(ref_sig), Delay10/1
  LimitPulseWidth11/1(ref_sig_limit) -> Relational Operator11/2
  Delay9/1 -> Switch28/3
  Delay10/1 -> Switch31/3
  U11_norm/1 -> Switch31/1
  Constant26/1 -> Switch33/3
  Switch30/1 -> Switch29/1
  LimitPulseWidth10/1(ref_sig_limit) -> Relational Operator10/2
  Switch33/1 -> Switch32/1
  Switch28/1 -> LimitPulseWidth9/1(ref_sig), Delay9/1
  Relational Operator10/1 -> Switch33/2
  Demux9/1 -> S19/1
  Relational Operator9/1 -> Switch30/2
  U12_norm/1 -> Switch34/1
  Delay11/1 -> Switch34/3
  PWM_en_AXI/1 -> PWM_en_rd_AXI/1, HDL Counter2/1, Switch35/2, Switch32/2, Switch29/2, Switch26/2, Switch23/2, Switch20/2, Switch17/2, Switch14/2, Switch11/2, Switch5/2, Switch4/2, Switch3/2
  Demux10/2 -> S22/1
  Constant23/1 -> Switch36/1
  Switch29/1 -> Demux9/1
  LimitPulseWidth9/1(ref_sig_limit) -> Relational Operator9/2
  Switch32/1 -> Demux10/1
  Constant22/1 -> Switch36/3
  Switch36/1 -> Switch35/1
  Demux9/2 -> S20/1
  Demux10/1 -> S21/1

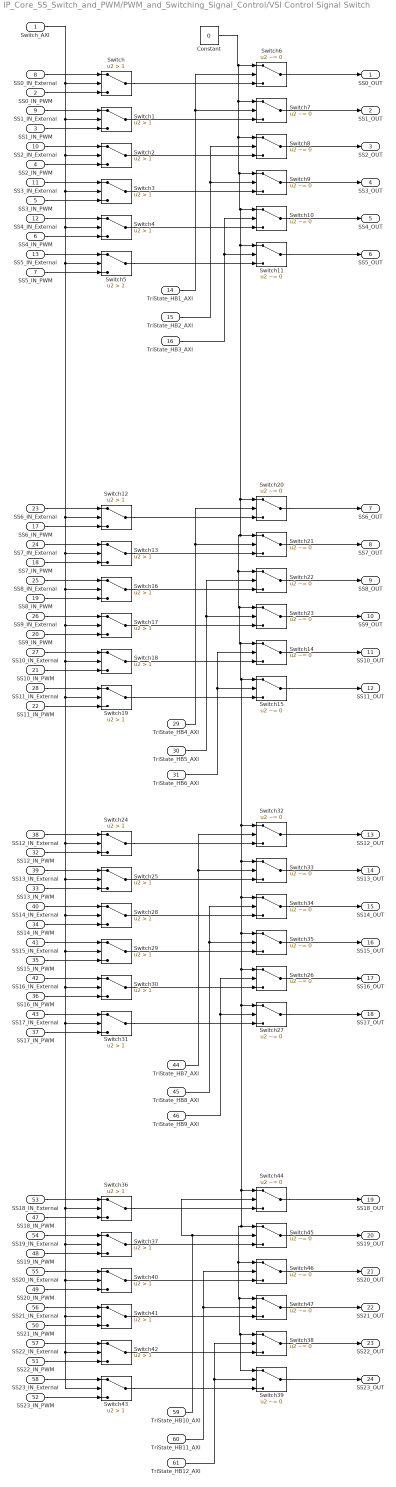
== system IP_Core_SS_Switch_and_PWM/PWM_and_Switching_Signal_Control/VSI Control Signal Switch ==
  Switch_AXI : Inport
  SS0_IN_PWM : Inport  Port=2
  SS1_IN_PWM : Inport  Port=3
  SS2_IN_PWM : Inport  Port=4
  SS3_IN_PWM : Inport  Port=5
  SS4_IN_PWM : Inport  Port=6
  SS5_IN_PWM : Inport  Port=7
  SS0_IN_External : Inport  Port=8
  SS1_IN_External : Inport  Port=9
  SS2_IN_External : Inport  Port=10
  SS3_IN_External : Inport  Port=11
  SS4_IN_External : Inport  Port=12
  SS5_IN_External : Inport  Port=13
  TriState_HB1_AXI : Inport  Port=14
  TriState_HB2_AXI : Inport  Port=15
  TriState_HB3_AXI : Inport  Port=16
  SS6_IN_PWM : Inport  Port=17
  SS7_IN_PWM : Inport  Port=18
  SS8_IN_PWM : Inport  Port=19
  SS9_IN_PWM : Inport  Port=20
  SS10_IN_PWM : Inport  Port=21
  SS11_IN_PWM : Inport  Port=22
  SS6_IN_External : Inport  Port=23
  SS7_IN_External : Inport  Port=24
  SS8_IN_External : Inport  Port=25
  SS9_IN_External : Inport  Port=26
  SS10_IN_External : Inport  Port=27
  SS11_IN_External : Inport  Port=28
  TriState_HB4_AXI : Inport  Port=29
  TriState_HB5_AXI : Inport  Port=30
  TriState_HB6_AXI : Inport  Port=31
  SS12_IN_PWM : Inport  Port=32
  SS13_IN_PWM : Inport  Port=33
  SS14_IN_PWM : Inport  Port=34
  SS15_IN_PWM : Inport  Port=35
  SS16_IN_PWM : Inport  Port=36
  SS17_IN_PWM : Inport  Port=37
  SS12_IN_External : Inport  Port=38
  SS13_IN_External : Inport  Port=39
  SS14_IN_External : Inport  Port=40
  SS15_IN_External : Inport  Port=41
  SS16_IN_External : Inport  Port=42
  SS17_IN_External : Inport  Port=43
  TriState_HB7_AXI : Inport  Port=44
  TriState_HB8_AXI : Inport  Port=45
  TriState_HB9_AXI : Inport  Port=46
  SS18_IN_PWM : Inport  Port=47
  SS19_IN_PWM : Inport  Port=48
  SS20_IN_PWM : Inport  Port=49
  SS21_IN_PWM : Inport  Port=50
  SS22_IN_PWM : Inport  Port=51
  SS23_IN_PWM : Inport  Port=52
  SS18_IN_External : Inport  Port=53
  SS19_IN_External : Inport  Port=54
  SS20_IN_External : Inport  Port=55
  SS21_IN_External : Inport  Port=56
  SS22_IN_External : Inport  Port=57
  SS23_IN_External : Inport  Port=58
  TriState_HB10_AXI : Inport  Port=59
  TriState_HB11_AXI : Inport  Port=60
  TriState_HB12_AXI : Inport  Port=61
  Constant : Constant  Value=0  OutDataTypeStr=boolean  SampleTime=T_FPGA_clk
  Switch{,1..5,12..13,16..19,24..25,28..31,36..37,40..43} (24 alike) : Switch  Criteria=u2 > Threshold  Threshold=1
  Switch{6..11,14..15,20..23,26..27,32..35,38..39,44..47} (24 alike) : Switch  Criteria=u2 ~= 0  Threshold=1
  SS0_OUT : Outport  VectorParamsAs1DForOutWhenUnconnected=off
  SS1_OUT : Outport  Port=2  VectorParamsAs1DForOutWhenUnconnected=off
  SS2_OUT : Outport  Port=3  VectorParamsAs1DForOutWhenUnconnected=off
  SS3_OUT : Outport  Port=4  VectorParamsAs1DForOutWhenUnconnected=off
  SS4_OUT : Outport  Port=5  VectorParamsAs1DForOutWhenUnconnected=off
  SS5_OUT : Outport  Port=6  VectorParamsAs1DForOutWhenUnconnected=off
  SS6_OUT : Outport  Port=7  VectorParamsAs1DForOutWhenUnconnected=off
  SS7_OUT : Outport  Port=8  VectorParamsAs1DForOutWhenUnconnected=off
  SS8_OUT : Outport  Port=9  VectorParamsAs1DForOutWhenUnconnected=off
  SS9_OUT : Outport  Port=10  VectorParamsAs1DForOutWhenUnconnected=off
  SS10_OUT : Outport  Port=11  VectorParamsAs1DForOutWhenUnconnected=off
  SS11_OUT : Outport  Port=12  VectorParamsAs1DForOutWhenUnconnected=off
  SS12_OUT : Outport  Port=13  VectorParamsAs1DForOutWhenUnconnected=off
  SS13_OUT : Outport  Port=14  VectorParamsAs1DForOutWhenUnconnected=off
  SS14_OUT : Outport  Port=15  VectorParamsAs1DForOutWhenUnconnected=off
  SS15_OUT : Outport  Port=16  VectorParamsAs1DForOutWhenUnconnected=off
  SS16_OUT : Outport  Port=17  VectorParamsAs1DForOutWhenUnconnected=off
  SS17_OUT : Outport  Port=18  VectorParamsAs1DForOutWhenUnconnected=off
  SS18_OUT : Outport  Port=19  VectorParamsAs1DForOutWhenUnconnected=off
  SS19_OUT : Outport  Port=20  VectorParamsAs1DForOutWhenUnconnected=off
  SS20_OUT : Outport  Port=21  VectorParamsAs1DForOutWhenUnconnected=off
  SS21_OUT : Outport  Port=22  VectorParamsAs1DForOutWhenUnconnected=off
  SS22_OUT : Outport  Port=23  VectorParamsAs1DForOutWhenUnconnected=off
  SS23_OUT : Outport  Port=24  VectorParamsAs1DForOutWhenUnconnected=off
  wires:
  Switch5/1 -> Switch11/3
  Switch/1 -> Switch6/3
  Switch3/1 -> Switch9/3
  Switch2/1 -> Switch8/3
  Switch1/1 -> Switch7/3
  Switch4/1 -> Switch10/3
  SS0_IN_PWM/1 -> Switch/3
  SS0_IN_External/1 -> Switch/1
  SS1_IN_External/1 -> Switch1/1
  SS1_IN_PWM/1 -> Switch1/3
  SS2_IN_External/1 -> Switch2/1
  SS2_IN_PWM/1 -> Switch2/3
  SS3_IN_External/1 -> Switch3/1
  SS3_IN_PWM/1 -> Switch3/3
  SS4_IN_External/1 -> Switch4/1
  SS4_IN_PWM/1 -> Switch4/3
  SS5_IN_External/1 -> Switch5/1
  SS5_IN_PWM/1 -> Switch5/3
  Switch11/1 -> SS5_OUT/1
  Switch10/1 -> SS4_OUT/1
  Switch9/1 -> SS3_OUT/1
  Switch8/1 -> SS2_OUT/1
  Switch7/1 -> SS1_OUT/1
  Switch6/1 -> SS0_OUT/1
  Switch23/1 -> SS9_OUT/1
  Switch20/1 -> SS6_OUT/1
  Switch22/1 -> SS8_OUT/1
  Switch13/1 -> Switch21/3
  Switch15/1 -> SS11_OUT/1
  Switch21/1 -> SS7_OUT/1
  Switch14/1 -> SS10_OUT/1
  SS7_IN_PWM/1 -> Switch13/3
  SS6_IN_PWM/1 -> Switch12/3
  Switch19/1 -> Switch15/3
  SS11_IN_External/1 -> Switch19/1
  SS9_IN_External/1 -> Switch17/1
  SS10_IN_PWM/1 -> Switch18/3
  SS8_IN_PWM/1 -> Switch16/3
  SS10_IN_External/1 -> Switch18/1
  Switch17/1 -> Switch23/3
  SS6_IN_External/1 -> Switch12/1
  SS8_IN_External/1 -> Switch16/1
  SS9_IN_PWM/1 -> Switch17/3
  Switch18/1 -> Switch14/3
  Switch12/1 -> Switch20/3
  Switch16/1 -> Switch22/3
  SS7_IN_External/1 -> Switch13/1
  Switch35/1 -> SS15_OUT/1
  Switch32/1 -> SS12_OUT/1
  Switch34/1 -> SS14_OUT/1
  Switch25/1 -> Switch33/3
  Switch27/1 -> SS17_OUT/1
  Switch33/1 -> SS13_OUT/1
  Switch26/1 -> SS16_OUT/1
  SS13_IN_PWM/1 -> Switch25/3
  SS12_IN_PWM/1 -> Switch24/3
  Switch31/1 -> Switch27/3
  SS17_IN_External/1 -> Switch31/1
  SS15_IN_External/1 -> Switch29/1
  SS16_IN_PWM/1 -> Switch30/3
  SS14_IN_PWM/1 -> Switch28/3
  SS16_IN_External/1 -> Switch30/1
  Switch29/1 -> Switch35/3
  SS12_IN_External/1 -> Switch24/1
  SS14_IN_External/1 -> Switch28/1
  SS15_IN_PWM/1 -> Switch29/3
  Switch30/1 -> Switch26/3
  Switch24/1 -> Switch32/3
  Switch28/1 -> Switch34/3
  SS13_IN_External/1 -> Switch25/1
  Constant/1 -> Switch20/1, Switch32/1, Switch44/1, Switch39/1, Switch38/1, Switch47/1, Switch46/1, Switch45/1, Switch27/1, Switch26/1, Switch35/1, Switch34/1, Switch33/1, Switch15/1, Switch14/1, Switch23/1, Switch22/1, Switch21/1, Switch11/1, Switch10/1, Switch9/1, Switch8/1, Switch7/1, Switch6/1
  Switch47/1 -> SS21_OUT/1
  Switch44/1 -> SS18_OUT/1
  Switch46/1 -> SS20_OUT/1
  Switch37/1 -> Switch45/3
  Switch39/1 -> SS23_OUT/1
  Switch45/1 -> SS19_OUT/1
  Switch38/1 -> SS22_OUT/1
  SS19_IN_PWM/1 -> Switch37/3
  SS18_IN_PWM/1 -> Switch36/3
  TriState_HB10_AXI/1 -> Switch44/2, Switch45/2
  Switch43/1 -> Switch39/3
  SS23_IN_External/1 -> Switch43/1
  SS21_IN_External/1 -> Switch41/1
  SS22_IN_PWM/1 -> Switch42/3
  SS20_IN_PWM/1 -> Switch40/3
  SS22_IN_External/1 -> Switch42/1
  Switch41/1 -> Switch47/3
  SS18_IN_External/1 -> Switch36/1
  SS20_IN_External/1 -> Switch40/1
  SS21_IN_PWM/1 -> Switch41/3
  Switch42/1 -> Switch38/3
  TriState_HB11_AXI/1 -> Switch46/2, Switch47/2
  Switch36/1 -> Switch44/3
  Switch40/1 -> Switch46/3
  TriState_HB12_AXI/1 -> Switch39/2, Switch38/2
  Switch_AXI/1 -> Switch4/2, Switch5/2, Switch12/2, Switch18/2, Switch19/2, Switch24/2, Switch30/2, Switch42/2, Switch43/2, Switch41/2, Switch40/2, Switch37/2, Switch36/2, Switch31/2, Switch29/2, Switch28/2, Switch25/2, Switch17/2, Switch16/2, Switch13/2, Switch3/2, Switch2/2, Switch1/2, Switch/2
  SS19_IN_External/1 -> Switch37/1
  TriState_HB1_AXI/1 -> Switch7/2, Switch6/2
  TriState_HB2_AXI/1 -> Switch9/2, Switch8/2
  TriState_HB3_AXI/1 -> Switch11/2, Switch10/2
  SS11_IN_PWM/1 -> Switch19/3
  TriState_HB4_AXI/1 -> Switch21/2, Switch20/2
  TriState_HB5_AXI/1 -> Switch23/2, Switch22/2
  TriState_HB6_AXI/1 -> Switch15/2, Switch14/2
  SS17_IN_PWM/1 -> Switch31/3
  TriState_HB7_AXI/1 -> Switch33/2, Switch32/2
  TriState_HB8_AXI/1 -> Switch35/2, Switch34/2
  TriState_HB9_AXI/1 -> Switch27/2, Switch26/2
  SS23_IN_PWM/1 -> Switch43/3

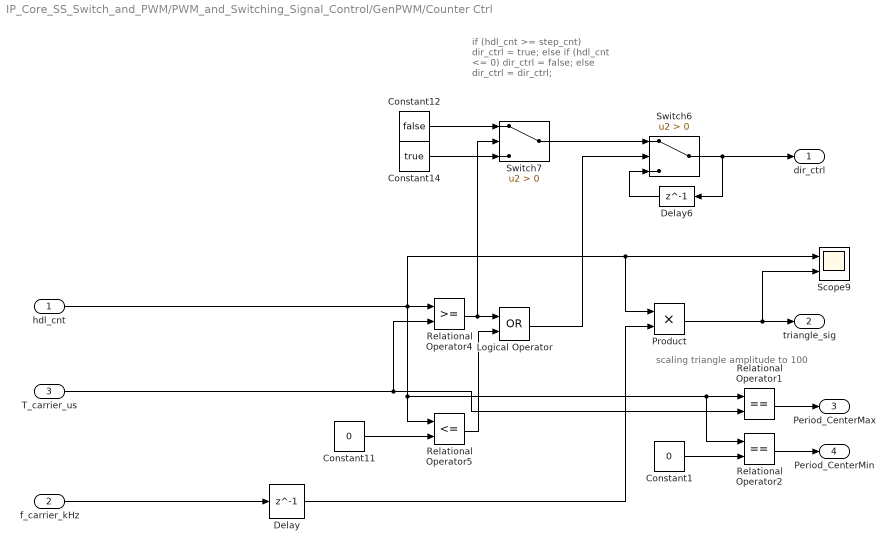
== system IP_Core_SS_Switch_and_PWM/PWM_and_Switching_Signal_Control/GenPWM/Counter Ctrl ==
  note: if (hdl_cnt >= step_cnt)
      | 	dir_ctrl = true;
      | else if (hdl_cnt <= 0)
      | 	dir_ctrl = false;
      | else
      | 	dir_ctrl = dir_ctrl;
  note: scaling triangle amplitude to 100
  hdl_cnt : Inport
  f_carrier_kHz : Inport  Port=2
  T_carrier_us : Inport  Port=3
  Constant1 : Constant  Value=0  OutDataTypeStr=fixdt(0,20,0)  SampleTime=T_FPGA_clk
  Constant11 : Constant  Value=0  OutDataTypeStr=fixdt(0,20,0)  SampleTime=T_FPGA_clk
  Constant12 : Constant  Value=false  SampleTime=T_FPGA_clk
  Constant14 : Constant  Value=true  SampleTime=T_FPGA_clk
  Delay : Delay  DelayLength=1
  Delay6 : Delay  DelayLength=1
  Logical Operator : Logic  Operator=OR  AllPortsSameDT=off  OutDataTypeStr=boolean
  Product : Product  OutDataTypeStr=fixdt(0,18,17)
  Relational Operator1 : RelationalOperator  Operator===  OutDataTypeStr=boolean  RndMeth=Nearest
  Relational Operator2 : RelationalOperator  Operator===  OutDataTypeStr=boolean  RndMeth=Nearest
  Relational Operator4 : RelationalOperator  OutDataTypeStr=boolean  RndMeth=Nearest
  Relational Operator5 : RelationalOperator  Operator=<=  OutDataTypeStr=boolean  RndMeth=Nearest
  Scope9 : Scope  NumInputPorts=2
  Switch6 : Switch  Criteria=u2 > Threshold
  Switch7 : Switch  Criteria=u2 > Threshold
  dir_ctrl : Outport  VectorParamsAs1DForOutWhenUnconnected=off
  triangle_sig : Outport  Port=2  VectorParamsAs1DForOutWhenUnconnected=off
  Period_CenterMax : Outport  Port=3  VectorParamsAs1DForOutWhenUnconnected=off
  Period_CenterMin : Outport  Port=4  VectorParamsAs1DForOutWhenUnconnected=off
  wires:
  hdl_cnt/1 -> Relational Operator2/1, Relational Operator1/1, Relational Operator5/1, Relational Operator4/1, Product/1, Scope9/1
  Switch6/1 -> Delay6/1, dir_ctrl/1
  Relational Operator4/1 -> Switch7/2, Logical Operator/1
  Relational Operator5/1 -> Logical Operator/2
  Constant11/1 -> Relational Operator5/2
  Logical Operator/1 -> Switch6/2
  Switch7/1 -> Switch6/1
  Constant12/1 -> Switch7/1
  Constant14/1 -> Switch7/3
  Delay6/1 -> Switch6/3
  T_carrier_us/1 -> Relational Operator4/2, Relational Operator1/2
  Product/1 -> triangle_sig/1, Scope9/2
  f_carrier_kHz/1 -> Delay/1
  Delay/1 -> Product/2
  Relational Operator1/1 -> Period_CenterMax/1
  Relational Operator2/1 -> Period_CenterMin/1
  Constant1/1 -> Relational Operator2/2

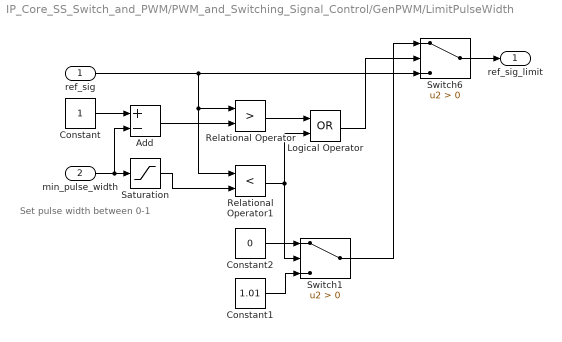
== system IP_Core_SS_Switch_and_PWM/PWM_and_Switching_Signal_Control/GenPWM/LimitPulseWidth ==
  note: Set pulse width between 0-1
  ref_sig : Inport
  min_pulse_width : Inport  Port=2
  Add : Sum  Inputs=+-  OutDataTypeStr=Inherit: Same as first input
  Constant : Constant  OutDataTypeStr=fixdt(1,18,16)  SampleTime=T_FPGA_clk
  Constant1 : Constant  Value=1.01  OutDataTypeStr=fixdt(1,18,16)  SampleTime=T_FPGA_clk
  Constant2 : Constant  Value=0  OutDataTypeStr=fixdt(1,18,16)  SampleTime=T_FPGA_clk
  Logical Operator : Logic  Operator=OR  AllPortsSameDT=off  OutDataTypeStr=boolean
  Relational Operator : RelationalOperator  Operator=>  OutDataTypeStr=boolean  RndMeth=Nearest
  Relational Operator1 : RelationalOperator  Operator=<  OutDataTypeStr=boolean  RndMeth=Nearest
  Saturation : Saturate  UpperLimit=1  LowerLimit=0  OutDataTypeStr=fixdt(1,18,16)
  Switch1 : Switch  Criteria=u2 > Threshold
  Switch6 : Switch  Criteria=u2 > Threshold
  ref_sig_limit : Outport  VectorParamsAs1DForOutWhenUnconnected=off
  wires:
  Constant/1 -> Add/1
  min_pulse_width/1 -> Add/2, Saturation/1
  Add/1 -> Relational Operator/2
  ref_sig/1 -> Switch6/3, Relational Operator/1, Relational Operator1/1
  Relational Operator/1 -> Logical Operator/1
  Relational Operator1/1 -> Logical Operator/2, Switch1/2
  Logical Operator/1 -> Switch6/2
  Constant1/1 -> Switch1/3
  Switch1/1 -> Switch6/1
  Constant2/1 -> Switch1/1
  Switch6/1 -> ref_sig_limit/1
  Saturation/1 -> Relational Operator1/2

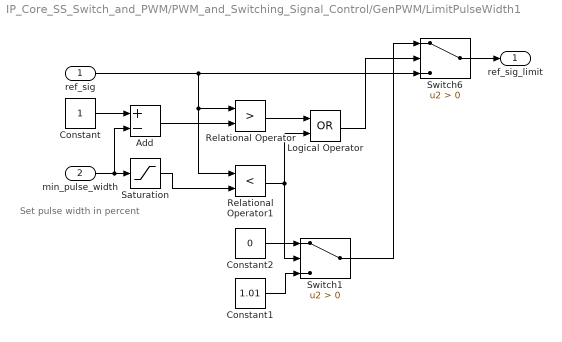
== system IP_Core_SS_Switch_and_PWM/PWM_and_Switching_Signal_Control/GenPWM/LimitPulseWidth1 ==
  note: Set pulse width in percent
  ref_sig : Inport
  min_pulse_width : Inport  Port=2
  Add : Sum  Inputs=+-  OutDataTypeStr=Inherit: Same as first input
  Constant : Constant  OutDataTypeStr=fixdt(1,18,16)  SampleTime=T_FPGA_clk
  Constant1 : Constant  Value=1.01  OutDataTypeStr=fixdt(1,18,16)  SampleTime=T_FPGA_clk
  Constant2 : Constant  Value=0  OutDataTypeStr=fixdt(1,18,16)  SampleTime=T_FPGA_clk
  Logical Operator : Logic  Operator=OR  AllPortsSameDT=off  OutDataTypeStr=boolean
  Relational Operator : RelationalOperator  Operator=>  OutDataTypeStr=boolean  RndMeth=Nearest
  Relational Operator1 : RelationalOperator  Operator=<  OutDataTypeStr=boolean  RndMeth=Nearest
  Saturation : Saturate  UpperLimit=1  LowerLimit=0  OutDataTypeStr=fixdt(1,18,16)
  Switch1 : Switch  Criteria=u2 > Threshold
  Switch6 : Switch  Criteria=u2 > Threshold
  ref_sig_limit : Outport  VectorParamsAs1DForOutWhenUnconnected=off
  wires:
  Constant/1 -> Add/1
  min_pulse_width/1 -> Add/2, Saturation/1
  Add/1 -> Relational Operator/2
  ref_sig/1 -> Switch6/3, Relational Operator/1, Relational Operator1/1
  Relational Operator/1 -> Logical Operator/1
  Relational Operator1/1 -> Logical Operator/2, Switch1/2
  Logical Operator/1 -> Switch6/2
  Constant1/1 -> Switch1/3
  Switch1/1 -> Switch6/1
  Constant2/1 -> Switch1/1
  Switch6/1 -> ref_sig_limit/1
  Saturation/1 -> Relational Operator1/2
